simulink model "TestSimulink2"  (R2017b)
settings: Solver=VariableStepAuto  StartTime=0.0  StopTime=20  RelTol=1e-3
undefined symbols (not defined in the file): A, C1, C2, C3, H11, H12, H21, H22, H23, H32, H33, K1, K2, K3, M11, M12, M21, M22, M23, M32, M33, N, n
settings Model: Creator=Nicola  LastModifiedBy=Nicola

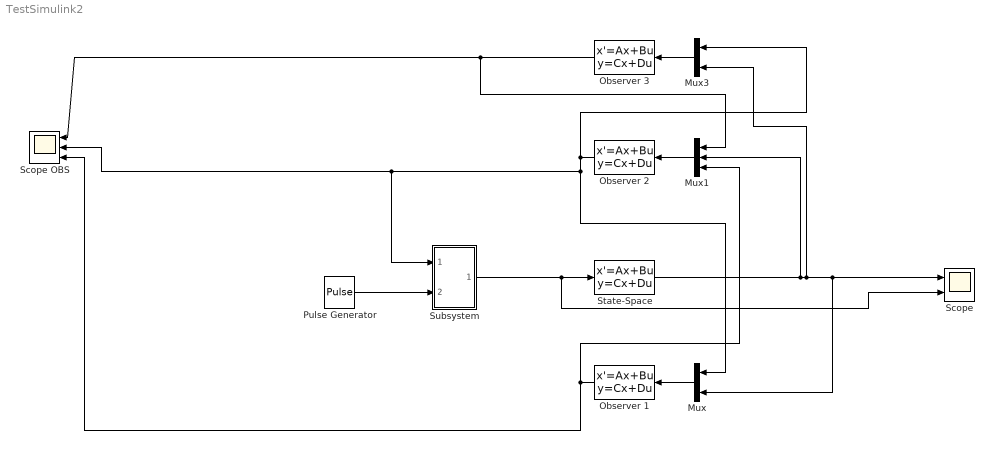
== system TestSimulink2 ==
  Mux : Mux  Inputs=2
  Mux1 : Mux  Inputs=3
  Mux3 : Mux  Inputs=2
  Observer 1 : StateSpace  A=H11  B=[H12 K1*C1]  C=[M11]  D=[M12 N]  InitialCondition=0
  Observer 2 : StateSpace  A=H22  B=[H23 K2*C2 H21]  C=[M22]  D=[M23 N M21]  InitialCondition=0
  Observer 3 : StateSpace  A=H33  B=[H32 K3*C3]  C=[M33]  D=[M32 N]  InitialCondition=0
  Pulse Generator : DiscretePulseGenerator  PulseType=Time based  Period=10  PulseWidth=10
  Scope : Scope  NumInputPorts=2
  Scope OBS : Scope  NumInputPorts=3
  State-Space : StateSpace  A=A  B=eye(n)  C=eye(n)  D=zeros(n,n)  InitialCondition=0
  Subsystem : Subsystem
  wires:
  State-Space/1 -> Mux1/2, Scope/1, Mux/2, Mux3/2
  Observer 1/1 -> Scope OBS/3, Mux1/3
  Mux/1 -> Observer 1/1
  Mux1/1 -> Observer 2/1
  Mux3/1 -> Observer 3/1
  Observer 3/1 -> Mux1/1, Scope OBS/1
  Observer 2/1 -> Subsystem/1(In1), Scope OBS/2, Mux/1, Mux3/1
  Subsystem/1(Out1) -> Scope/2, State-Space/1
  Pulse Generator/1 -> Subsystem/2(In2)

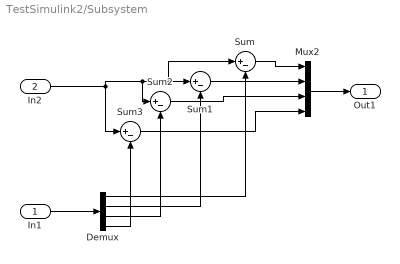
== system TestSimulink2/Subsystem ==
  In1 : Inport
  In2 : Inport  Port=2
  Demux : Demux
  Mux2 : Mux
  Sum{,1..3} (4 alike) : Sum  Inputs=|+-
  Out1 : Outport
  wires:
  In1/1 -> Demux/1
  Demux/4 -> Sum3/2
  Sum1/1 -> Mux2/2
  Demux/1 -> Sum/2
  Demux/2 -> Sum1/2
  Mux2/1 -> Out1/1
  Demux/3 -> Sum2/2
  In2/1 -> Sum2/1, Sum1/1, Sum/1, Sum3/1
  Sum/1 -> Mux2/1
  Sum3/1 -> Mux2/4
  Sum2/1 -> Mux2/3
